simulink model "dev_sim_lineal_kalman"  (R2019b)
settings: Solver=VariableStepAuto  StartTime=0.0  StopTime=500.0  RelTol=1e-3
values from neighbouring files (symbols this model uses):
  A_0 = eval(A_0)    [modelo.m]    (also in modelo_var.m; parametros.mat = [0 -3.26931291643 0 0.71460251427 0 0 0 0 1 -0.0325743287495)
  B_0 = eval(B_0)    [modelo.m]    (also in modelo_var.m; parametros.mat = [0 0 0 0 0 0 1190.47619048 0 0 0 0 0 ... (16 elements, 8x2)])
  C_0 = eval(C_0)    [modelo.m]    (also in modelo_var.m; parametros.mat = [1 0 0 0 0 1 0 0 0 0 0 0 ... (16 elements, 2x8)])
  D_0 = eval(D_0)    [modelo.m]    (also in modelo_var.m; parametros.mat = [0  0; 0  0])
  L = Ec-Ep    [modelo.m]    (also in modelo_var.m)
settings Model: Creator=tronc  LastModifiedBy=tronc

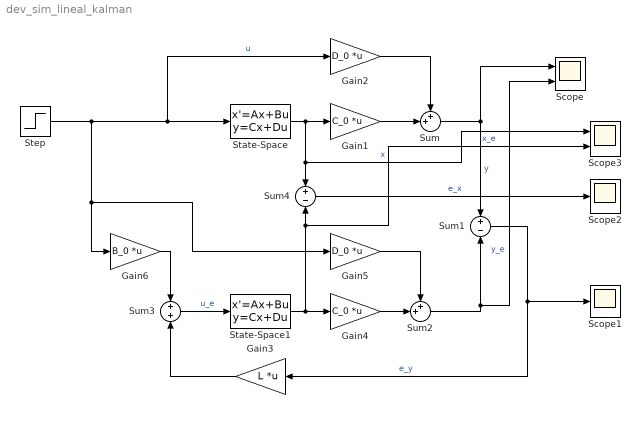
== system dev_sim_lineal_kalman ==
  Gain1 : Gain  Gain=C_0  Multiplication=Matrix(K*u)
  Gain2 : Gain  Gain=D_0  Multiplication=Matrix(K*u)
  Gain3 : Gain  Gain=L  Multiplication=Matrix(K*u)
  Gain4 : Gain  Gain=C_0  Multiplication=Matrix(K*u)
  Gain5 : Gain  Gain=D_0  Multiplication=Matrix(K*u)
  Gain6 : Gain  Gain=B_0  Multiplication=Matrix(K*u)
  Scope : Scope  NumInputPorts=2
  Scope1 : Scope
  Scope2 : Scope
  Scope3 : Scope  NumInputPorts=2
  State-Space : StateSpace  A=A_0  B=B_0  C=eye(8)  D=zeros(8,2)  InitialCondition=[1 1 0 0 0 0 0 0]
  State-Space1 : StateSpace  A=A_0  B=eye(8)  C=eye(8)  D=zeros(8)  InitialCondition=[-1 -1 0 0 0 0 0 0]
  Step : Step  Before=[0 0]  After=[0 0]  SampleTime=0
  Sum : Sum  Inputs=++|
  Sum1 : Sum  Inputs=+|-
  Sum2 : Sum  Inputs=++|
  Sum3 : Sum  Inputs=+|+
  Sum4 : Sum  Inputs=+|-
  wires:
  State-Space/1 -> Scope3/1, Sum4/1, Gain1/1  "x"
  Sum/1 -> Sum1/1, Scope/1  "y"
  Gain2/1 -> Sum/1
  Gain1/1 -> Sum/2
  Step/1 -> State-Space/1, Gain2/1, Gain5/1, Gain6/1  "u"
  State-Space1/1 -> Scope3/2, Sum4/2, Gain4/1  "x_e"
  Gain4/1 -> Sum2/2
  Gain5/1 -> Sum2/1
  Sum2/1 -> Scope/2, Sum1/2  "y_e"
  Sum1/1 -> Gain3/1, Scope1/1  "e_y"
  Sum3/1 -> State-Space1/1  "u_e"
  Gain3/1 -> Sum3/2
  Gain6/1 -> Sum3/1
  Sum4/1 -> Scope2/1  "e_x"
